simulink model "twa_parallel_pc104"  (R2016a)
settings: Solver=ode8  StartTime=0.0  StopTime=inf  FixedStep=dt  RelTol=1e-3
PreLoadFcn:
  | addpath('d:\Projects\TwistedWireActuator\TWA_parallel_control\init_func')
InitFcn:
  | init_main_twa
  | init_scopes
  | init_twa_homing
  | init_twa_wires
undefined symbols (not defined in the file or in its folder): b_in_w, dt, enc_res_vec, f_in_w, gear_rat_vec, Kd, Kd_mu, Ki, Ki_mu, Kp, Kp_mu, m_in_w, meas_flex_pos, N_velocity, p_in_m, pid_mode, qmacro_nom, res_rate_param, reset_integ, Signed, t_in_w, twa_gamma, twa_offset, use_twa, vel_filter_coeffs, velmex_pitch, wire_delta, wire_rad
libraries: xpcsensoraylib x7, slrtlib x6, simulink x4, dspswit3 x1
CloseFcn:
  | rtwprivate ssgencode ModelCloseRequest acrochordidae_v1
settings Model: Creator=Roger  LastModifiedBy=ahronoez
settings SolverCC: EnableConcurrentExecution=on
settings DataIOCC: SaveFormat=StructureWithTime  SignalLoggingSaveFormat=ModelDataLogs
settings OptimizationCC: BlockReduction=off  OptimizeBlockIOStorage=off  BufferReuse=off  GlobalBufferReuse=off  ExpressionFolding=off  ExpressionDepthLimit=2147483647  LocalBlockOutputs=off  InitFltsAndDblsToZero=on
settings DebuggingCC: UnderspecifiedInitializationDetection=Classic  MergeDetectMultiDrivingBlocksExec=none  SolverPrmCheckMsg=warning  FcnCallInpInsideContextMsg=UseLocalSettings  StateNameClashWarn=warning
settings HardwareCC: ProdBitPerPointer=32  ProdLargestAtomicFloat=None  ProdWordSize=32  ProdLongLongMode=on  ProdHWDeviceType=Generic->32-bit x86 compatible
settings ModelReferenceCC: PropagateSignalLabelsOutOfModel=off
settings SFSimCC: SimParseCustomCode=off
settings RTWCC: SystemTargetFile=slrt.tlc  TLCOptions=-aSLRTFTZOFF=1  TemplateMakefile=slrt_default_tmf  Description=Simulink Real-Time  GenerateReport=on  RTWCompilerOptimization=Custom  RTWCustomCompilerOptimizations=/arch-IA32
settings SimulinkRealTimeCC: xPCisDownloadable=off
settings ConfigComp: CovModelRefEnable=Off

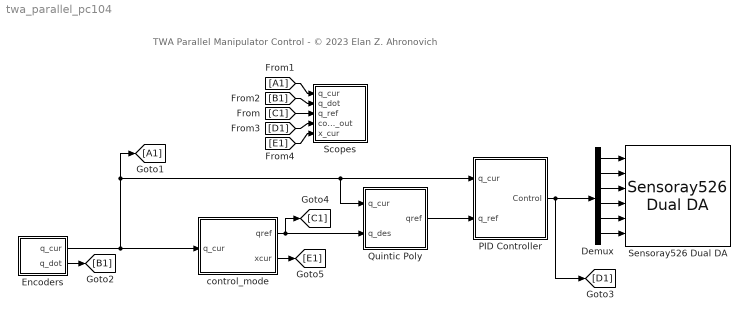
== system twa_parallel_pc104 ==
  note: TWA Parallel Manipulator Control - © 2023 Elan Z. Ahronovich
  Demux : Demux  Outputs=6
  Encoders : Subsystem
  PID Controller : Subsystem
  Quintic Poly : Subsystem
  Scopes : Subsystem
  "Sensoray526 Dual DA " : xpcsensoraylib/D//A/Sensoray526 Dual DA   channel1=[1 2 3 4]  reset1=[0]  initial1=[0]  channel2=[1 2]  reset2=[0]  initial2=[0]  sampletime=dt  baseaddress1=0x2c0  baseaddress2=0x340
  control_mode : Subsystem
  wires:
  PID Controller/1(Control) -> [D1], Demux/1
  Demux/1 -> "Sensoray526 Dual DA "/1
  Demux/2 -> "Sensoray526 Dual DA "/2
  Demux/3 -> "Sensoray526 Dual DA "/3
  Demux/4 -> "Sensoray526 Dual DA "/4
  Demux/5 -> "Sensoray526 Dual DA "/5
  Demux/6 -> "Sensoray526 Dual DA "/6
  Encoders/1(q_cur) -> PID Controller/1(q_cur), Quintic Poly/1(q_cur), [A1], control_mode/1(q_cur)
  Encoders/2(q_dot) -> [B1]
  Quintic Poly/1(qref) -> PID Controller/2(q_ref)
  [C1] -> Scopes/3(q_ref)
  [A1] -> Scopes/1(q_cur)
  [B1] -> Scopes/2(q_dot)
  [D1] -> Scopes/4(control_out)
  [E1] -> Scopes/5(x_cur)
  control_mode/1(qref) -> Quintic Poly/2(q_des), [C1]
  control_mode/2(xcur) -> [E1]

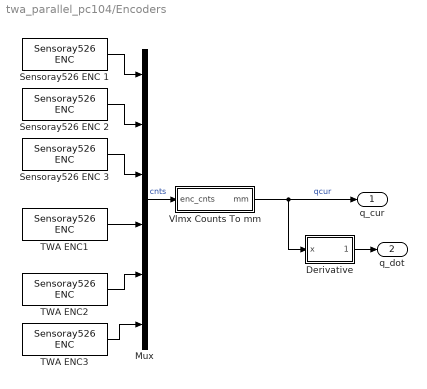
== system twa_parallel_pc104/Encoders ==
  Derivative : Subsystem
  Mux : Mux  Inputs=6
  Sensoray526 ENC 1 : xpcsensoraylib/Encoder/Sensoray526 ENC   channel=1  index=None  resetval=0  initval=0  range=Signed +-2^23  speed=4x  sampletime=dt  baseaddress=0x2c0
  Sensoray526 ENC 2 : xpcsensoraylib/Encoder/Sensoray526 ENC   channel=2  index=None  resetval=0  initval=0  range=Signed +-2^23  speed=4x  sampletime=dt  baseaddress=0x2c0
  Sensoray526 ENC 3 : xpcsensoraylib/Encoder/Sensoray526 ENC   channel=3  index=None  resetval=0  initval=0  range=Signed +-2^23  speed=4x  sampletime=dt  baseaddress=0x2c0
  TWA ENC1 : xpcsensoraylib/Encoder/Sensoray526 ENC   channel=4  index=None  resetval=0  initval=0  range=Signed +-2^23  speed=4x  sampletime=dt  baseaddress=0x2c0
  TWA ENC2 : xpcsensoraylib/Encoder/Sensoray526 ENC   channel=1  index=None  resetval=0  initval=0  range=Signed +-2^23  speed=4x  sampletime=dt  baseaddress=0x340
  TWA ENC3 : xpcsensoraylib/Encoder/Sensoray526 ENC   channel=2  index=None  resetval=0  initval=0  range=Signed +-2^23  speed=4x  sampletime=dt  baseaddress=0x340
  Vlmx Counts To mm : Subsystem
  q_cur : Outport
  q_dot : Outport  Port=2
  wires:
  Sensoray526 ENC 1/1 -> Mux/1
  Sensoray526 ENC 2/1 -> Mux/2
  Sensoray526 ENC 3/1 -> Mux/3
  Vlmx Counts To mm/1(mm) -> Derivative/1(x), q_cur/1  "qcur"
  Mux/1 -> Vlmx Counts To mm/1(enc_cnts)  "cnts"
  Derivative/1(x_dot) -> q_dot/1
  TWA ENC1/1 -> Mux/4
  TWA ENC2/1 -> Mux/5
  TWA ENC3/1 -> Mux/6

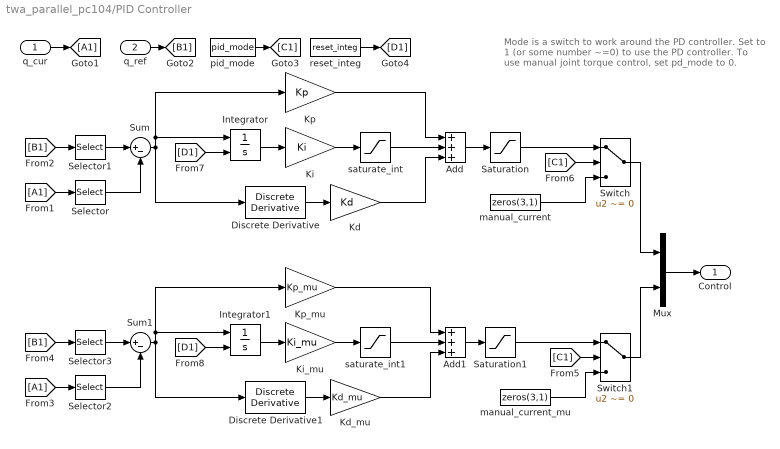
== system twa_parallel_pc104/PID Controller ==
  note: Mode is a switch to work around the PD controller.
      | Set to 1 (or some number ~=0) to use the PD
      | controller. To use manual joint torque control, set
      | pd_mode to 0.
  q_cur : Inport
  q_ref : Inport  Port=2
  Add : Sum  Inputs=+++
  Add1 : Sum  Inputs=+++
  Discrete Derivative : simulink/Discrete/Discrete Derivative  gainval=1.0  ICPrevScaledInput=0.0  InputProcessing=Inherited  OutMin=[]  OutMax=[]  OutDataType=fixdt(1, 16)  OutScaling=2^-10  DoSatur=off
  Discrete Derivative1 : simulink/Discrete/Discrete Derivative  gainval=1.0  ICPrevScaledInput=0.0  InputProcessing=Inherited  OutMin=[]  OutMax=[]  OutDataType=fixdt(1, 16)  OutScaling=2^-10  DoSatur=off
  Integrator : Integrator  ExternalReset=rising
  Integrator1 : Integrator  ExternalReset=rising
  Kd : Gain  Gain=Kd
  Kd_mu : Gain  Gain=Kd_mu
  Ki : Gain  Gain=Ki
  Ki_mu : Gain  Gain=Ki_mu
  Kp : Gain  Gain=Kp
  Kp_mu : Gain  Gain=Kp_mu
  Mux : Mux  Inputs=2
  Saturation : Saturate  UpperLimit=[10,10,10]  LowerLimit=-1*[10,10,10]  LinearizeAsGain=off
  Saturation1 : Saturate  UpperLimit=5*ones(3,1)  LowerLimit=-5*ones(3,1)  LinearizeAsGain=off
  Selector : Selector  InputPortWidth=6  IndexOptions=Index vector (dialog)  Indices=[1 2 3]  OutputSizes=1
  Selector1 : Selector  InputPortWidth=6  IndexOptions=Index vector (dialog)  Indices=[1 2 3]  OutputSizes=1
  Selector2 : Selector  InputPortWidth=6  IndexOptions=Index vector (dialog)  Indices=[4 5 6]  OutputSizes=1
  Selector3 : Selector  InputPortWidth=6  IndexOptions=Index vector (dialog)  Indices=[4 5 6]  OutputSizes=1
  Sum : Sum  Inputs=|+-
  Sum1 : Sum  Inputs=|+-
  Switch : Switch  Criteria=u2 ~= 0
  Switch1 : Switch  Criteria=u2 ~= 0
  manual_current : Constant  Value=zeros(3,1)  SampleTime=-1
  manual_current_mu : Constant  Value=zeros(3,1)  SampleTime=-1
  pid_mode : Constant  Value=pid_mode  SampleTime=-1
  reset_integ : Constant  Value=reset_integ  SampleTime=-1
  saturate_int : Saturate  UpperLimit=[5,5,5]  LowerLimit=-1*[5,5,5]  LinearizeAsGain=off
  saturate_int1 : Saturate  UpperLimit=2.5*ones(3,1)  LowerLimit=-2.5*ones(3,1)  LinearizeAsGain=off  SampleTime=dt
  Control : Outport
  wires:
  Kp/1 -> Add/1
  Kd/1 -> Add/3
  Add/1 -> Saturation/1
  Saturation/1 -> Switch/1
  manual_current/1 -> Switch/3
  Ki/1 -> saturate_int/1
  saturate_int/1 -> Add/2
  Discrete Derivative/1 -> Kd/1
  Integrator/1 -> Ki/1
  Sum/1 -> Kp/1, Integrator/1, Discrete Derivative/1
  Kp_mu/1 -> Add1/1
  Kd_mu/1 -> Add1/3
  Add1/1 -> Saturation1/1
  Saturation1/1 -> Switch1/1
  manual_current_mu/1 -> Switch1/3
  Ki_mu/1 -> saturate_int1/1
  saturate_int1/1 -> Add1/2
  Discrete Derivative1/1 -> Kd_mu/1
  Integrator1/1 -> Ki_mu/1
  Sum1/1 -> Kp_mu/1, Integrator1/1, Discrete Derivative1/1
  q_cur/1 -> [A1]
  q_ref/1 -> [B1]
  [A1] -> Selector/1
  [B1] -> Selector1/1
  [A1] -> Selector2/1
  [B1] -> Selector3/1
  pid_mode/1 -> [C1]
  [C1] -> Switch1/2
  [C1] -> Switch/2
  Mux/1 -> Control/1
  Switch/1 -> Mux/1
  Switch1/1 -> Mux/2
  Selector1/1 -> Sum/1
  Selector/1 -> Sum/2
  Selector3/1 -> Sum1/1
  Selector2/1 -> Sum1/2
  reset_integ/1 -> [D1]
  [D1] -> Integrator/2
  [D1] -> Integrator1/2

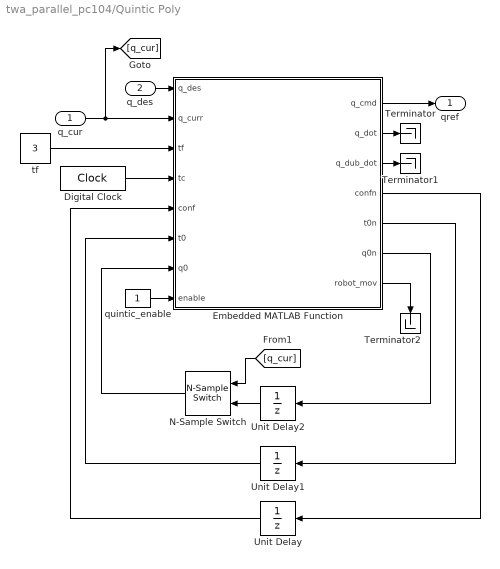
== system twa_parallel_pc104/Quintic Poly ==
  q_cur : Inport
  q_des : Inport  Port=2
  Digital Clock : DigitalClock  SampleTime=dt
  Embedded MATLAB Function : MATLAB Function  TreatAsAtomicUnit=on
  N-Sample Switch : dspswit3/N-Sample Switch  N=1  reset=off  TriggerType=Rising edge  Ts=dt
  Terminator : Terminator
  Terminator1 : Terminator
  Terminator2 : Terminator
  Unit Delay : UnitDelay  SampleTime=-1
  Unit Delay1 : UnitDelay  SampleTime=-1
  Unit Delay2 : UnitDelay  InitialCondition=zeros(6,1)  SampleTime=-1
  quintic_enable : Constant  SampleTime=-1
  tf : Constant  Value=3  SampleTime=-1
  qref : Outport
  wires:
  Embedded MATLAB Function/4(confn) -> Unit Delay/1
  Unit Delay/1 -> Embedded MATLAB Function/5(conf)
  Embedded MATLAB Function/5(t0n) -> Unit Delay1/1
  Embedded MATLAB Function/6(q0n) -> Unit Delay2/1
  Unit Delay1/1 -> Embedded MATLAB Function/6(t0)
  Digital Clock/1 -> Embedded MATLAB Function/4(tc)
  q_des/1 -> Embedded MATLAB Function/1(q_des)
  tf/1 -> Embedded MATLAB Function/3(tf)
  quintic_enable/1 -> Embedded MATLAB Function/8(enable)
  Embedded MATLAB Function/2(q_dot) -> Terminator/1
  Embedded MATLAB Function/3(q_dub_dot) -> Terminator1/1
  N-Sample Switch/1 -> Embedded MATLAB Function/7(q0)
  Unit Delay2/1 -> N-Sample Switch/2
  [q_cur] -> N-Sample Switch/1
  Embedded MATLAB Function/7(robot_mov) -> Terminator2/1
  Embedded MATLAB Function/1(q_cmd) -> qref/1
  q_cur/1 -> Embedded MATLAB Function/2(q_curr), [q_cur]

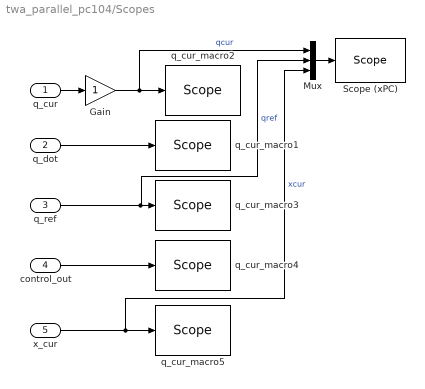
== system twa_parallel_pc104/Scopes ==
  q_cur : Inport
  q_dot : Inport  Port=2
  q_ref : Inport  Port=3
  control_out : Inport  Port=4
  x_cur : Inport  Port=5
  Gain : Gain
  Mux : Mux  Inputs=3
  "Scope (xPC) " : slrtlib/Displays and Logging/Scope   scopeno=6  scopetype=File  autostart=off  viewmode=Graphical redraw  formatstr='%15.6f'  grid=on  ylimits=[0,0]  nosamples=3  noprepostsamples=0  interleave=1  triggermode=FreeRun  triggersignal=1  trigsignalfromport=off  triggerlevel=0.0  triggerslope=Either  triggerscope=1  triggersample=0  filename=robot.dat  mode=Lazy  writesize=512  autorestart=on  dynamicfilemode=off  maxwritefilesize=512*1024^2
  q_cur_macro1 : slrtlib/Displays and Logging/Scope   scopeno=2  scopetype=Target  autostart=on  viewmode=Numerical  formatstr=qd_format  grid=on  ylimits=[0,0]  nosamples=25  noprepostsamples=0  interleave=1  triggermode=FreeRun  triggersignal=1  trigsignalfromport=off  triggerlevel=0.0  triggerslope=Either  triggerscope=1  triggersample=0  filename=data.dat  mode=Lazy  writesize=512  autorestart=off  dynamicfilemode=off  maxwritefilesize=512*1024^2
  q_cur_macro2 : slrtlib/Displays and Logging/Scope   scopeno=1  scopetype=Target  autostart=on  viewmode=Numerical  formatstr=q_format  grid=on  ylimits=[0,0]  nosamples=3  noprepostsamples=0  interleave=1  triggermode=FreeRun  triggersignal=1  trigsignalfromport=off  triggerlevel=0.0  triggerslope=Either  triggerscope=1  triggersample=0  filename=data.dat  mode=Lazy  writesize=512  autorestart=off  dynamicfilemode=off  maxwritefilesize=512*1024^2
  q_cur_macro3 : slrtlib/Displays and Logging/Scope   scopeno=3  scopetype=Target  autostart=on  viewmode=Numerical  formatstr=qdes_format  grid=on  ylimits=[0,0]  nosamples=25  noprepostsamples=0  interleave=1  triggermode=FreeRun  triggersignal=1  trigsignalfromport=off  triggerlevel=0.0  triggerslope=Either  triggerscope=1  triggersample=0  filename=data.dat  mode=Lazy  writesize=512  autorestart=off  dynamicfilemode=off  maxwritefilesize=512*1024^2
  q_cur_macro4 : slrtlib/Displays and Logging/Scope   scopeno=4  scopetype=Target  autostart=on  viewmode=Numerical  formatstr=qcmd_format  grid=on  ylimits=[0,0]  nosamples=25  noprepostsamples=0  interleave=1  triggermode=FreeRun  triggersignal=1  trigsignalfromport=off  triggerlevel=0.0  triggerslope=Either  triggerscope=1  triggersample=0  filename=data.dat  mode=Lazy  writesize=512  autorestart=off  dynamicfilemode=off  maxwritefilesize=512*1024^2
  q_cur_macro5 : slrtlib/Displays and Logging/Scope   scopeno=5  scopetype=Target  autostart=on  viewmode=Numerical  formatstr=xcur_format  grid=on  ylimits=[0,0]  nosamples=25  noprepostsamples=0  interleave=1  triggermode=FreeRun  triggersignal=1  trigsignalfromport=off  triggerlevel=0.0  triggerslope=Either  triggerscope=1  triggersample=0  filename=data.dat  mode=Lazy  writesize=512  autorestart=off  dynamicfilemode=off  maxwritefilesize=512*1024^2
  wires:
  q_ref/1 -> Mux/2, q_cur_macro3/1  "qref"
  control_out/1 -> q_cur_macro4/1
  x_cur/1 -> Mux/3, q_cur_macro5/1  "xcur"
  q_dot/1 -> q_cur_macro1/1
  q_cur/1 -> Gain/1
  Gain/1 -> Mux/1, q_cur_macro2/1  "qcur"
  Mux/1 -> "Scope (xPC) "/1

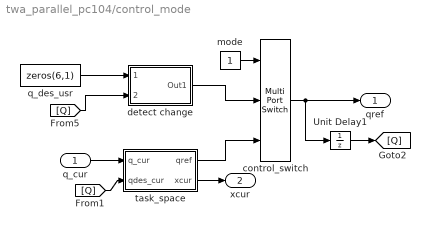
== system twa_parallel_pc104/control_mode ==
  q_cur : Inport
  Unit Delay1 : UnitDelay  InitialCondition=zeros(6,1)  SampleTime=-1
  control_switch : MultiPortSwitch  Inputs=2  DiagnosticForDefault=Warning
  detect change : Subsystem
  mode : Constant  SampleTime=-1
  q_des_usr : Constant  Value=zeros(6,1)  SampleTime=-1
  task_space : Subsystem
  qref : Outport
  xcur : Outport  Port=2
  wires:
  mode/1 -> control_switch/1
  control_switch/1 -> Unit Delay1/1, qref/1
  [Q] -> detect change/2(q_des_cur)
  detect change/1(Out1) -> control_switch/2
  q_des_usr/1 -> detect change/1(q_des_usr)
  q_cur/1 -> task_space/1(q_cur)
  task_space/2(xcur) -> xcur/1
  Unit Delay1/1 -> [Q]
  [Q] -> task_space/2(qdes_cur)
  task_space/1(qref) -> control_switch/3

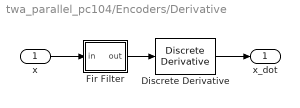
== system twa_parallel_pc104/Encoders/Derivative ==
  x : Inport
  Discrete Derivative : simulink/Discrete/Discrete Derivative  gainval=1.0  ICPrevScaledInput=0.0  InputProcessing=Inherited  OutMin=[]  OutMax=[]  OutDataType=fixdt(1, 16)  OutScaling=2^-10  DoSatur=off
  Fir Filter : Subsystem
  x_dot : Outport
  wires:
  Discrete Derivative/1 -> x_dot/1
  x/1 -> Fir Filter/1(in)
  Fir Filter/1(out) -> Discrete Derivative/1

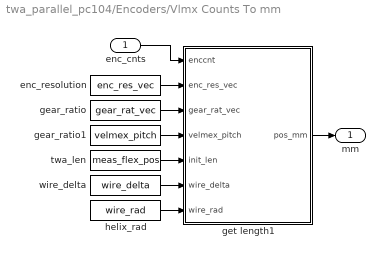
== system twa_parallel_pc104/Encoders/Vlmx Counts To mm ==
  enc_cnts : Inport
  enc_resolution : Constant  Value=enc_res_vec  SampleTime=-1
  gear_ratio : Constant  Value=gear_rat_vec  SampleTime=-1
  gear_ratio1 : Constant  Value=velmex_pitch  SampleTime=-1
  get length1 : MATLAB Function  TreatAsAtomicUnit=on
  helix_rad : Constant  Value=wire_rad  SampleTime=-1
  twa_len : Constant  Value=meas_flex_pos  SampleTime=-1
  wire_delta : Constant  Value=wire_delta  SampleTime=-1
  mm : Outport
  wires:
  helix_rad/1 -> get length1/7(wire_rad)
  wire_delta/1 -> get length1/6(wire_delta)
  twa_len/1 -> get length1/5(init_len)
  enc_resolution/1 -> get length1/2(enc_res_vec)
  gear_ratio/1 -> get length1/3(gear_rat_vec)
  enc_cnts/1 -> get length1/1(enccnt)
  get length1/1(pos_mm) -> mm/1
  gear_ratio1/1 -> get length1/4(velmex_pitch)

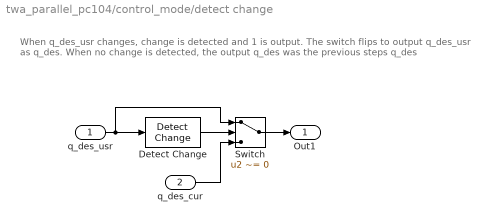
== system twa_parallel_pc104/control_mode/detect change ==
  note: When q_des_usr changes, change is detected and 1 is output.
      | The switch flips to output q_des_usr as q_des. When no change is detected, the output
      | q_des was the previous steps q_des
  q_des_usr : Inport
  q_des_cur : Inport  Port=2
  Detect Change : simulink/Logic and Bit Operations/Detect Change  vinit=zeros(6,1)  InputProcessing=Inherited  OutDataTypeStr=uint8
  Switch : Switch  Criteria=u2 ~= 0
  Out1 : Outport
  wires:
  Detect Change/1 -> Switch/2
  q_des_usr/1 -> Switch/1, Detect Change/1
  Switch/1 -> Out1/1
  q_des_cur/1 -> Switch/3

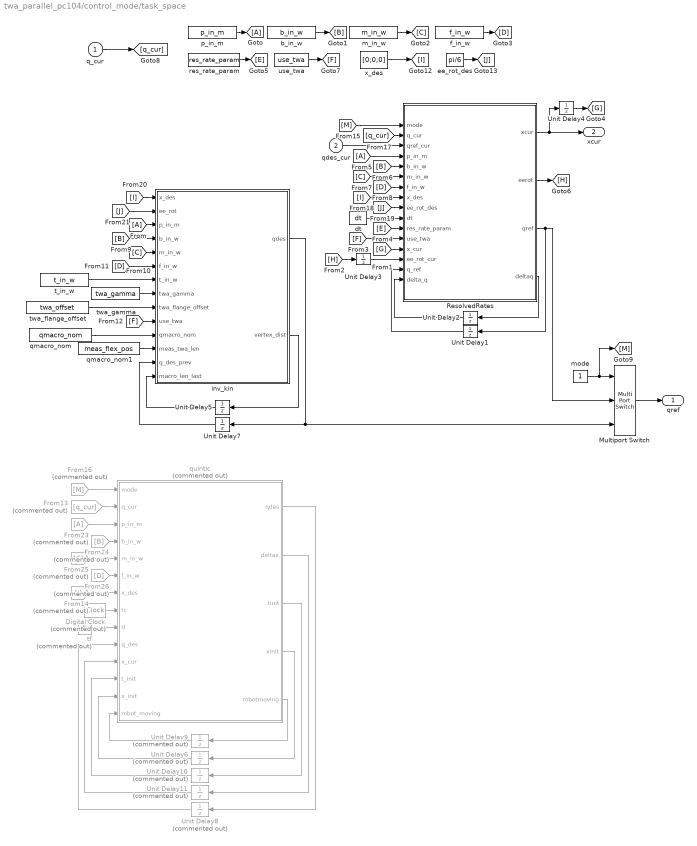
== system twa_parallel_pc104/control_mode/task_space ==
  q_cur : Inport
  qdes_cur : Inport  Port=2
  Digital Clock : DigitalClock  Commented=on  SampleTime=dt
  From13 : From  Commented=on  GotoTag=q_cur
  From14 : From  Commented=on  GotoTag=I
  From16 : From  Commented=on  GotoTag=M
  From23 : From  Commented=on
  From24 : From  Commented=on  GotoTag=B
  From25 : From  Commented=on  GotoTag=C
  From26 : From  Commented=on  GotoTag=D
  Multiport Switch : MultiPortSwitch  Inputs=2  DiagnosticForDefault=Warning
  ResolvedRates : MATLAB Function  TreatAsAtomicUnit=on
  Unit Delay1 : UnitDelay  InitialCondition=[0;0;0;0;0;0]  SampleTime=-1
  Unit Delay10 : UnitDelay  Commented=on  SampleTime=dt
  Unit Delay11 : UnitDelay  Commented=on  InitialCondition=[0;0;0]  SampleTime=dt
  Unit Delay2 : UnitDelay  InitialCondition=[0;0;0;0;0;0]  SampleTime=-1
  Unit Delay3 : UnitDelay  InitialCondition=pi/6  SampleTime=-1
  Unit Delay4 : UnitDelay  InitialCondition=[0;0;0]  SampleTime=-1
  Unit Delay5 : UnitDelay  InitialCondition=qmacro_nom  SampleTime=-1
  Unit Delay6 : UnitDelay  Commented=on  InitialCondition=[0;0;0]  SampleTime=dt
  Unit Delay7 : UnitDelay  InitialCondition=[0;0;0;0;0;0]  SampleTime=-1
  Unit Delay8 : UnitDelay  Commented=on  InitialCondition=zeros(6,1)  SampleTime=dt
  Unit Delay9 : UnitDelay  Commented=on  SampleTime=dt
  b_in_w : Constant  Value=b_in_w  SampleTime=-1
  dt : Constant  Value=dt  SampleTime=-1
  ee_rot_des : Constant  Value=pi/6  SampleTime=-1
  f_in_w : Constant  Value=f_in_w  SampleTime=-1
  inv_kin : MATLAB Function  TreatAsAtomicUnit=on
  m_in_w : Constant  Value=m_in_w  SampleTime=-1
  mode : Constant  SampleTime=-1
  p_in_m : Constant  Value=p_in_m  SampleTime=-1
  qmacro_nom : Constant  Value=qmacro_nom  SampleTime=-1
  qmacro_nom1 : Constant  Value=meas_flex_pos  SampleTime=-1
  quintic : MATLAB Function  Commented=on  TreatAsAtomicUnit=on
  res_rate_param : Constant  Value=res_rate_param  SampleTime=-1
  t_in_w : Constant  Value=t_in_w  SampleTime=-1
  tf : Constant  Commented=on  Value=5  SampleTime=dt
  twa_flange_offset : Constant  Value=twa_offset  SampleTime=-1
  twa_gamma : Constant  Value=twa_gamma  SampleTime=-1
  use_twa : Constant  Value=use_twa  SampleTime=-1
  x_des : Constant  Value=[0;0;0]  SampleTime=-1
  qref : Outport
  xcur : Outport  Port=2
  wires:
  p_in_m/1 -> [A]
  b_in_w/1 -> [B]
  m_in_w/1 -> [C]
  f_in_w/1 -> [D]
  dt/1 -> ResolvedRates/10(dt)
  qdes_cur/1 -> ResolvedRates/3(qref_cur)
  Unit Delay1/1 -> ResolvedRates/15(q_ref)
  ResolvedRates/3(qref) -> Unit Delay1/1, Multiport Switch/2
  [E] -> ResolvedRates/11(res_rate_param)
  res_rate_param/1 -> [E]
  ResolvedRates/2(eerot) -> [H]
  [H] -> Unit Delay3/1
  ResolvedRates/1(xcur) -> Unit Delay4/1, xcur/1
  [F] -> ResolvedRates/12(use_twa)
  use_twa/1 -> [F]
  ResolvedRates/4(deltaq) -> Unit Delay2/1
  Unit Delay2/1 -> ResolvedRates/16(delta_q)
  [A] -> inv_kin/3(p_in_m)
  [B] -> inv_kin/4(b_in_w)
  [C] -> inv_kin/5(m_in_w)
  [D] -> inv_kin/6(f_in_w)
  q_cur/1 -> [q_cur]
  [q_cur] -> ResolvedRates/2(q_cur)
  x_des/1 -> [I]
  ee_rot_des/1 -> [J]
  [I] -> ResolvedRates/8(x_des)
  [J] -> ResolvedRates/9(ee_rot_des)
  [I] -> inv_kin/1(x_des)
  [J] -> inv_kin/2(ee_rot)
  twa_gamma/1 -> inv_kin/8(twa_gamma)
  twa_flange_offset/1 -> inv_kin/9(twa_flange_offset)
  t_in_w/1 -> inv_kin/7(t_in_w)
  [F] -> inv_kin/10(use_twa)
  Multiport Switch/1 -> qref/1
  inv_kin/1(qdes) -> Multiport Switch/3, Unit Delay7/1
  Unit Delay7/1 -> inv_kin/13(q_des_prev)
  qmacro_nom/1 -> inv_kin/11(qmacro_nom)
  Unit Delay4/1 -> [G]
  Unit Delay3/1 -> ResolvedRates/14(ee_rot_cur)
  [G] -> ResolvedRates/13(x_cur)
  [A] -> ResolvedRates/4(p_in_m)
  [B] -> ResolvedRates/5(b_in_w)
  [C] -> ResolvedRates/6(m_in_w)
  [D] -> ResolvedRates/7(f_in_w)
  qmacro_nom1/1 -> inv_kin/12(meas_twa_len)
  inv_kin/2(vertex_dist) -> Unit Delay5/1
  Unit Delay5/1 -> inv_kin/14(macro_len_last)
  mode/1 -> [M], Multiport Switch/1
  [M] -> ResolvedRates/1(mode)
  From14/1 -> quintic/7(x_des)
  From23/1 -> quintic/3(p_in_m)
  From25/1 -> quintic/5(m_in_w)
  From24/1 -> quintic/4(b_in_w)
  From26/1 -> quintic/6(f_in_w)
  Digital Clock/1 -> quintic/8(tc)
  tf/1 -> quintic/9(tf)
  quintic/4(xinit) -> Unit Delay6/1
  quintic/5(robotmoving) -> Unit Delay9/1
  Unit Delay6/1 -> quintic/13(x_init)
  Unit Delay9/1 -> quintic/14(robot_moving)
  quintic/3(tinit) -> Unit Delay10/1
  Unit Delay10/1 -> quintic/12(t_init)
  quintic/2(deltax) -> Unit Delay11/1
  Unit Delay11/1 -> quintic/11(x_cur)
  quintic/1(qdes) -> Unit Delay8/1
  Unit Delay8/1 -> quintic/10(q_des)
  From13/1 -> quintic/2(q_cur)
  From16/1 -> quintic/1(mode)

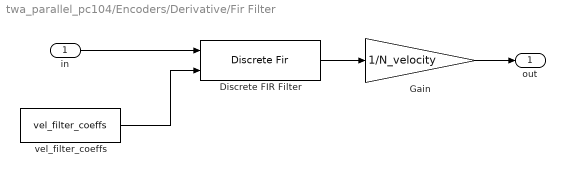
== system twa_parallel_pc104/Encoders/Derivative/Fir Filter ==
  in : Inport
  Discrete FIR Filter : DiscreteFir  CoefSource=Input port  AccumDataTypeStr=Inherit: Same as product output
      settings: InputPortMap=u0,u1
  Gain : Gain  Gain=1/N_velocity
  vel_filter_coeffs : Constant  Value=vel_filter_coeffs  SampleTime=-1
  out : Outport
  wires:
  Discrete FIR Filter/1 -> Gain/1
  vel_filter_coeffs/1 -> Discrete FIR Filter/2
  Gain/1 -> out/1
  in/1 -> Discrete FIR Filter/1

== matlab function twa_parallel_pc104/control_mode/task_space/ResolvedRates ==
  data: xcur output; eerot output; mode input; q_cur input; qref_cur input; p_in_m input; b_in_w input; m_in_w input; f_in_w input; qref output; x_des input; ee_rot_des input; dt input; res_rate_param input; use_twa input; x_cur input; ee_rot_cur input; q_ref input; delta_q input; deltaq output
% using resolved rates with redundacny resolution to solve robot position
% elan ahronovich 08/2024

function [xcur,eerot,qref,deltaq] = redResRate(mode,q_cur,qref_cur,...
    p_in_m,b_in_w,m_in_w,f_in_w,x_des,ee_rot_des,...
    dt,res_rate_param,use_twa,x_cur,ee_rot_cur,q_ref,delta_q)

% initialize
qref = qref_cur;
eerot = ee_rot_cur;
deltaq = delta_q;

% if using inv kin to control robot position its a safe assumption from the
% perspective of resolved rates that the current position of the ee is the 
% requested desired position. This helps keep the resolved rates updated
% with the current robot position without relying on the resolved rates to 
% solve for it which will accumulate error over some time
if mode == 2
    xcur = x_des;
else
    xcur = x_cur;
end

% axis for jacobian definitions
z0 = [0 0 1]';

% rotation matrix
r_cur = [cos(ee_rot_cur) -sin(ee_rot_cur) 0;sin(ee_rot_cur) cos(ee_rot_cur) 0;0 0 1];

% moving platform vertex locations
p_in_w = x_cur*ones(1,3) + r_cur*p_in_m;

%% instantaneous direct kinematics jacobian
% vector from base vertex to moving platform vertex
n1hat = (p_in_w(:,1)-b_in_w(:,1))./norm(b_in_w(:,1) - p_in_w(:,1));
n2hat = (p_in_w(:,2)-b_in_w(:,2))./norm(b_in_w(:,2) - p_in_w(:,2));
n3hat = (p_in_w(:,3)-b_in_w(:,3))./norm(b_in_w(:,3) - p_in_w(:,3));

a13 = z0'*(cross(r_cur*p_in_m(:,1),n1hat));
a23 = z0'*(cross(r_cur*p_in_m(:,2),n2hat));
a33 = z0'*(cross(r_cur*p_in_m(:,3),n3hat));

idk_jac = [n1hat(1,1) n1hat(2,1) a13; ...
    n2hat(1,1) n2hat(2,1) a23; ...
    n3hat(1,1) n3hat(2,1) a33];

%% instantaneous inverse kinematics jacobian
% micro actuator (TWA) lengths
q1_mu = norm(b_in_w(:,1) - m_in_w(:,1));
q2_mu = norm(b_in_w(:,2) - m_in_w(:,2));
q3_mu = norm(b_in_w(:,3) - m_in_w(:,3));

% vector from base vertex to twa motor attachment point
l1_hat = (m_in_w(:,1) - b_in_w(:,1)) ./ norm(m_in_w(:,1) - b_in_w(:,1));
l2_hat = (m_in_w(:,2) - b_in_w(:,2)) ./ norm(m_in_w(:,2) - b_in_w(:,2));
l3_hat = (m_in_w(:,3) - b_in_w(:,3)) ./ norm(m_in_w(:,3) - b_in_w(:,3));

% distance from micro actuator attachmnet point (m_i) to flexure rotation
%center (f_i)
a1 = norm(m_in_w(:,1) - f_in_w(:,1));
a2 = norm(m_in_w(:,2) - f_in_w(:,2));
a3 = norm(m_in_w(:,3) - f_in_w(:,3));

% distance from flexure rotation center (f_i) to base vertex
c1 = norm(b_in_w(:,1)-f_in_w(:,1));
c2 = norm(b_in_w(:,2)-f_in_w(:,2));
c3 = norm(b_in_w(:,3)-f_in_w(:,3));

% term to paramterize angle between a_i and qimu, delta
h1 = (c1^2 - a1^2 - q1_mu^2)/(-2*a1*q1_mu);
h2 = (c2^2 - a2^2 - q2_mu^2)/(-2*a2*q2_mu);
h3 = (c3^2 - a3^2 - q3_mu^2)/(-2*a3*q3_mu);

% time derivatives
h1dot = (4*a1*q1_mu^2 + (c1^2 - a1^2 - q1_mu^2)*2*a1) / (4*a1^2*q1_mu^2);
h2dot = (4*a2*q2_mu^2 + (c2^2 - a2^2 - q2_mu^2)*2*a2) / (4*a2^2*q2_mu^2);
h3dot = (4*a3*q3_mu^2 + (c3^2 - a3^2 - q3_mu^2)*2*a3) / (4*a3^2*q3_mu^2);

e1 = n1hat' * l1_hat + q1_mu*h1dot/sqrt(1-h1^2) * n1hat' * cross(z0,l1_hat);
e2 = n2hat' * l2_hat + q2_mu*h2dot/sqrt(1-h2^2) * n2hat' * cross(z0,l2_hat);
e3 = n3hat' * l3_hat + q3_mu*h3dot/sqrt(1-h3^2) * n3hat' * cross(z0,l3_hat);

% micro motion instantaneous inverse kinematics jacobian
b_mu = [e1 0 0;...
    0 e2 0;...
    0 0 e3];

% macro motion instantaneous inverse kinematics jacobian
b_m = eye(3);

% combined macro-micro motion IIK jacobian
iik_jac = [b_m,b_mu];

% positional error
p_del = norm(x_des - x_cur);

% positional error direction vector
if p_del ~= 0
    p_ep_hat = (x_des-x_cur)/p_del;
else
    p_ep_hat = zeros(3,1);
end

%*
% This can probably be replaced with scalar angular difference that will
% always bout about me = [0 0 1]'
%*

% desired orientation angle rotation matrix and error roation matrix
r_des = [cos(ee_rot_des) -sin(ee_rot_des) 0;sin(ee_rot_des) cos(ee_rot_des) 0;0 0 1];
r_cur = [cos(ee_rot_cur) -sin(ee_rot_cur) 0;sin(ee_rot_cur) cos(ee_rot_cur) 0;0 0 1];
r_del = r_des * r_cur';

% orientational error angle and axis
theta_e = acos((trace(r_del)-1)/2);

% orientational error axis
if theta_e ~= 0
    me = (1/(2*sin(theta_e)))*[r_del(3,2)-r_del(2,3);...
        r_del(1,3)-r_del(3,1);...
        r_del(2,1)-r_del(1,2)];
else
    me = z0;
end

% error thresholds
p_eps = res_rate_param(1,1);
w_eps = res_rate_param(2,1);
p_eps_mu = res_rate_param(1,2);
w_eps_mu = res_rate_param(2,2);

% linear velocity
vmax = res_rate_param(3,1);
vmin = res_rate_param(4,1);
vmax_mu = res_rate_param(3,2);
vmin_mu = res_rate_param(4,2);

% rotational velocity
wmax = res_rate_param(5,1);
wmin = res_rate_param(6,1);
wmax_mu = res_rate_param(5,2);
wmin_mu = res_rate_param(6,2);

% convergence radius multiplier
p_lambda = res_rate_param(7,1);
w_lambda = res_rate_param(8,1);
p_lambda_mu = res_rate_param(7,2);
w_lambda_mu = res_rate_param(8,2);

if mode == 1
    if theta_e > w_eps || p_del > p_eps
        % linear velocity multiplier
        if p_del ~=0
            if p_del/p_eps <= p_lambda
                vdot = vmin + (((vmax-vmin)*(p_del-p_eps))/(p_eps*(p_lambda-1)));
            else
                vdot = vmax;
            end
        else
            vdot = 0;
        end
        
        % angular velocity multiplier
        if theta_e ~= 0
            if theta_e/w_eps <= w_lambda && theta_e ~= 0
                wdot = wmin + (((wmax-wmin)*(theta_e-w_eps))/(w_eps*(w_lambda-1)));
            else
                wdot = wmax;
            end
        else
            wdot = 0;
        end
        
        % xdot_des components
        v = vdot * p_ep_hat;
        w = wdot * me;
        
        % jacobian weight matrix for macro actuator preference
        w_mat = diag([ones(1,3),1e10*ones(1,3)]);
        
        % construct jacobian
        full_jac = (w_mat\iik_jac') / (iik_jac/w_mat*iik_jac') * idk_jac;
        
        % qdot des using inverse kinematics with redundancy
        qdot = full_jac * [v(1:2);w(3)];
        
        % new desired q values
        deltaq = qdot * dt;

        qref = q_ref + deltaq;
        
        % integrate current position
        xcur = x_cur + v * dt;
        eerot = ee_rot_cur + w(3) * dt;
        % now that the macro motion has converged we can use micro actuators
    elseif theta_e > w_eps_mu || p_del > p_eps_mu
        if use_twa
            %         qdes = qdes_cur;
            %         xcur = x_cur;
            %         eerot = ee_rot_cur;
            % same as macro, only iterate twa length if they have arrived at
            % last desired location
            % linear velocity multiplier
            if p_del ~=0
                if p_del/p_eps_mu <= p_lambda_mu
                    vdot = vmin_mu + (((vmax_mu-vmin_mu)*...
                        (p_del-p_eps_mu))/(p_eps_mu*(p_lambda_mu-1)));
                else
                    vdot = vmax_mu;
                end
            else
                vdot = 0;
            end
            
            % angular velocity multiplier
            if theta_e ~= 0
                if theta_e/w_eps_mu <= w_lambda_mu && theta_e ~= 0
                    wdot = wmin_mu + (((wmax_mu - wmin_mu)*...
                        (theta_e - w_eps_mu))/(w_eps_mu*(w_lambda_mu-1)));
                else
                    wdot = wmax_mu;
                end
            else
                wdot = 0;
            end
            
            % xdot_des components
            v = vdot * p_ep_hat;
            w = wdot * me;
            
            % jacobian weight matrix for micro actuator preference
            w_mat = diag([1e10*ones(1,3),ones(1,3)]);
            
            % construct jacobian
            full_jac = (w_mat\iik_jac') / (iik_jac/w_mat*iik_jac') * idk_jac;
            
            % qdot des using inverse kinematics with redundancy
            qdot = full_jac * [v(1:2,1);w(3,1)];
            
            % new desired q values
            deltaq = qdot * dt;
            qref = q_ref + deltaq;
            
            % integrate current position
            xcur = x_cur + (dt*v);
            eerot = ee_rot_cur + w(3) * dt;
        end
    end
end

end

== matlab function twa_parallel_pc104/control_mode/task_space/quintic ==
  data: qdes output; mode input; q_cur input; p_in_m input; b_in_w input; m_in_w input; f_in_w input; x_des input; tc input; tf input; q_des input; x_cur input; t_init input; x_init input; deltax output; tinit output; xinit output; robot_moving input; robotmoving output
% using resolved rates with redundacny resolution to solve robot position
% elan ahronovich 08/2024

function [qdes,deltax,tinit,xinit,robotmoving] = quintic(mode,q_cur,...
    p_in_m,b_in_w,m_in_w,f_in_w,x_des,...
    tc,tf,q_des,x_cur,t_init,x_init,robot_moving)

% initialize
qdes = q_des;
deltax = x_cur;
tinit = t_init;
xinit = x_init;
robotmoving = robot_moving;

if mode == 3; do_quintic = 1; else do_quintic =0; end

% axis for jacobian definitions
z0 = [0 0 1]';

% rotation matrix
ee_rot_cur = pi/6;
r_cur = [cos(ee_rot_cur) -sin(ee_rot_cur) 0;sin(ee_rot_cur) cos(ee_rot_cur) 0;0 0 1];

% moving platform vertex locations
p_in_w = x_cur*ones(1,3) + r_cur*p_in_m;

%% instantaneous direct kinematics jacobian
% vector from base vertex to moving platform vertex
n1hat = (p_in_w(:,1)-b_in_w(:,1))./norm(b_in_w(:,1) - p_in_w(:,1));
n2hat = (p_in_w(:,2)-b_in_w(:,2))./norm(b_in_w(:,2) - p_in_w(:,2));
n3hat = (p_in_w(:,3)-b_in_w(:,3))./norm(b_in_w(:,3) - p_in_w(:,3));

a13 = z0'*(cross(r_cur*p_in_m(:,1),n1hat));
a23 = z0'*(cross(r_cur*p_in_m(:,2),n2hat));
a33 = z0'*(cross(r_cur*p_in_m(:,3),n3hat));

idk_jac = [n1hat(1,1) n1hat(2,1) a13; ...
    n2hat(1,1) n2hat(2,1) a23; ...
    n3hat(1,1) n3hat(2,1) a33];

%% instantaneous inverse kinematics jacobian
% micro actuator (TWA) lengths
q1_mu = norm(b_in_w(:,1) - m_in_w(:,1));
q2_mu = norm(b_in_w(:,2) - m_in_w(:,2));
q3_mu = norm(b_in_w(:,3) - m_in_w(:,3));

% vector from base vertex to twa motor attachment point
l1_hat = (m_in_w(:,1) - b_in_w(:,1)) ./ norm(m_in_w(:,1) - b_in_w(:,1));
l2_hat = (m_in_w(:,2) - b_in_w(:,2)) ./ norm(m_in_w(:,2) - b_in_w(:,2));
l3_hat = (m_in_w(:,3) - b_in_w(:,3)) ./ norm(m_in_w(:,3) - b_in_w(:,3));

% distance from micro actuator attachmnet point (m_i) to flexure rotation
%center (f_i)
a1 = norm(m_in_w(:,1) - f_in_w(:,1));
a2 = norm(m_in_w(:,2) - f_in_w(:,2));
a3 = norm(m_in_w(:,3) - f_in_w(:,3));

% distance from flexure rotation center (f_i) to base vertex
c1 = norm(b_in_w(:,1)-f_in_w(:,1));
c2 = norm(b_in_w(:,2)-f_in_w(:,2));
c3 = norm(b_in_w(:,3)-f_in_w(:,3));

% term to paramterize angle between a_i and qimu, delta
h1 = (c1^2 - a1^2 - q1_mu^2)/(-2*a1*q1_mu);
h2 = (c2^2 - a2^2 - q2_mu^2)/(-2*a2*q2_mu);
h3 = (c3^2 - a3^2 - q3_mu^2)/(-2*a3*q3_mu);

% time derivatives
h1dot = (4*a1*q1_mu^2 + (c1^2 - a1^2 - q1_mu^2)*2*a1) / (4*a1^2*q1_mu^2);
h2dot = (4*a2*q2_mu^2 + (c2^2 - a2^2 - q2_mu^2)*2*a2) / (4*a2^2*q2_mu^2);
h3dot = (4*a3*q3_mu^2 + (c3^2 - a3^2 - q3_mu^2)*2*a3) / (4*a3^2*q3_mu^2);

e1 = n1hat' * l1_hat + q1_mu*h1dot/sqrt(1-h1^2) * n1hat' * cross(z0,l1_hat);
e2 = n2hat' * l2_hat + q2_mu*h2dot/sqrt(1-h2^2) * n2hat' * cross(z0,l2_hat);
e3 = n3hat' * l3_hat + q3_mu*h3dot/sqrt(1-h3^2) * n3hat' * cross(z0,l3_hat);

% micro motion instantaneous inverse kinematics jacobian
b_mu = [e1 0 0;...
    0 e2 0;...
    0 0 e3];

% macro motion instantaneous inverse kinematics jacobian
b_m = eye(3);

% combined macro-micro motion IIK jacobian
iik_jac = [b_m,b_mu];

% positional error
p_del = x_des - x_init;
w_del = norm(x_des(3,1) - x_init(3,1));

%
if do_quintic && norm(p_del) > 0
    if robot_moving
        t = tc - t_init;
        if t < tf
            eta = t/tf;
            a3 = 10*eta^3;
            a4 = -15*eta^4;
            a5 = 6*eta^5;
            
            % apply quintic polynomial on task space
            deltax = x_init + p_del*(a3+a4+a5);
            
            % redundancy weight matrix favoring velmex up to 50 microns
            % from destination
            if norm(p_del) > 0.050
                w_mat = diag([ones(1,3),1e10*ones(1,3)]);
               macro_motion = 1;
            else
                w_mat = diag([ones(1,3),1e10*ones(1,3)]);
                macro_motion = 0;
            end
            
            % construct jacobian
            full_jac = (w_mat\iik_jac') / (iik_jac/w_mat*iik_jac') * idk_jac;
            
            % deltaq ~ J * deltax
            deltaq = full_jac * deltax;
            
            % new desired q values
            if macro_motion
                % new desired q values
                qdes(1:3,1) = deltaq(1:3,1);
                qdes(4:6,1) = q_cur(4:6,1);
            else
                qdes(4:6,1) = deltaq(4:6,1);
                qdes(1:3,1) = q_cur(1:3,1);
            end
        else
            robotmoving = 0;
        end
    else
        qdes = q_cur;
        tinit = tc;
        xinit = x_cur;
        robotmoving = 1;
    end
end

end

== matlab function twa_parallel_pc104/Encoders/Vlmx Counts To mm/get length1 ==
  data: enccnt input; enc_res_vec input; gear_rat_vec input; velmex_pitch input; init_len input; wire_delta input; wire_rad input; pos_mm output
% this function converts encoder counts to mm
% elan ahronovich 09/2024

function pos_mm  = fcn(enccnt,enc_res_vec,gear_rat_vec,velmex_pitch,init_len,wire_delta,wire_rad)
% velmex slides
pos_mm1 = enccnt(1,1)*(1/enc_res_vec(1,1))*(1/gear_rat_vec(1,1))*velmex_pitch;
pos_mm2 = enccnt(2,1)*(1/enc_res_vec(2,1))*(1/gear_rat_vec(2,1))*velmex_pitch;
pos_mm3 = enccnt(3,1)*(1/enc_res_vec(3,1))*(1/gear_rat_vec(3,1))*velmex_pitch;

% twisted wire actuators
% convert counts to radians
theta_mu1 = enccnt(4,1)*(1/enc_res_vec(4,1))*(1/gear_rat_vec(4,1))*2*pi; %[radians]
theta_mu2 = enccnt(5,1)*(1/enc_res_vec(5,1))*(1/gear_rat_vec(5,1))*2*pi; %[radians]
theta_mu3 = enccnt(6,1)*(1/enc_res_vec(6,1))*(1/gear_rat_vec(6,1))*2*pi; %[radians]

% estimate length of helix. model cannot handle when motors return to zero
% for some reason, the motors will run off. force a constant solution for
% the length in this case
if theta_mu1 == 0
    twa_len1 = 0;
else
    twa_len1 = init_len(1,1)-sqrt(init_len(1,1)^2*(1+wire_delta(1,1))^2 - (theta_mu1^2*wire_rad(1,1)^2));
end

if theta_mu2 == 0
    twa_len2 = 0;
else
    twa_len2 = init_len(2,1)-sqrt(init_len(2,1)^2*(1+wire_delta(2,1))^2 - (theta_mu2^2*wire_rad(2,1)^2));
end

if theta_mu3 == 0
    twa_len3 = 0;
else
    twa_len3 = init_len(3,1)-sqrt(init_len(3,1)^2*(1+wire_delta(3,1))^2 - (theta_mu3^2*wire_rad(3,1)^2));
end

pos_mm = [pos_mm1;pos_mm2;pos_mm3;twa_len1;twa_len2;twa_len3];
end

== matlab function twa_parallel_pc104/control_mode/task_space/inv_kin ==
  data: qdes output; vertex_dist output; x_des input; ee_rot input; p_in_m input; b_in_w input; m_in_w input; f_in_w input; t_in_w input; twa_gamma input; twa_flange_offset input; use_twa input; qmacro_nom input; meas_twa_len input; q_des_prev input; macro_len_last input
% This function solves for the vertex positions of the base and moving
% platform for a given desired end effector position.
% elan ahronovich 07/2024

function [qdes,vertex_dist] = fcn(x_des,ee_rot,p_in_m,b_in_w,m_in_w,f_in_w,...
                                  t_in_w,twa_gamma,twa_flange_offset,use_twa,...
                                  qmacro_nom,meas_twa_len,q_des_prev,macro_len_last)

qdes = q_des_prev;
% des_micro_len = micro_len;

vertex_dist = macro_len_last;

% rotation matrix of moving frame about z-xis
rot_m2w = [cos(ee_rot) -sin(ee_rot) 0; sin(ee_rot) cos(ee_rot) 0; 0 0 1];

p_in_w = x_des*ones(1,3) + rot_m2w*p_in_m;

%%%%%%%%%%%%%%%%%%%%%%%%%%%%%%%%
%        Macro Actuator        %
%%%%%%%%%%%%%%%%%%%%%%%%%%%%%%%%

if ~use_twa
    vertex_dist = p_in_w - b_in_w;
    qdes(1,1) = norm(vertex_dist(:,1)) - norm(qmacro_nom(:,1));
    qdes(2,1) = norm(vertex_dist(:,2)) - norm(qmacro_nom(:,2));
    qdes(3,1) = norm(vertex_dist(:,3)) - norm(qmacro_nom(:,3));
end

%%%%%%%%%%%%%%%%%%%%%%%%%%%%%%%%
%       Micro Actuator         %
%%%%%%%%%%%%%%%%%%%%%%%%%%%%%%%%

if use_twa 
    % initial flexure bend
    beta_cmd = 0;
    
    % loop through each vertex
    for i = 1:3
        post_flex_angle = zeros(1,2);
        beta = zeros(1,2);
        
        % vector from flexure center to moving platform vertex
        rho_vec = p_in_w(:,i) - f_in_w(:,i);
        
        % distance between flexure and moving platform verteces
        rho = norm(rho_vec);
        
        % vector from flexure center to base vertex pre flexure rotation
        eta_vec = b_in_w(:,i) - f_in_w(:,i);
        
        % flexure angle at the start (e.g. 5 deg preload) in world frame
        pre_flex_angle = atan2(eta_vec(2,1),eta_vec(1,1));
        
        % magnitude of flexure swing-arm radius from flexure to base vertex
        eta = norm(eta_vec);
        
        % angle from world horizontal to the vector from the flexure
        % center to the platform vertex
        flexure_frame_rot_angle = atan2(rho_vec(2,1),rho_vec(1,1));
        
        % rotation matrix from flexure frame to world
        n = [0;0;1] ./ norm([0;0;1]);
        rot_f_2_w = expm(flexure_frame_rot_angle*[0 -n(3) n(2);n(3) 0 -n(1);n(2) n(1) 0]);
        
        % condition for acos solvability
        check = (norm(vertex_dist(:,i))^2-rho^2-eta^2)/(-2*rho*eta);
%         check = (des_macro_len(i,1)^2-rho^2-eta^2)/(-2*rho*eta);
        
        if check >= -1 && check <= 1
            % calculate angle between mf and fb vectors, lambda, with
            % law of cosines
            lambda = acos(check);
            
            % calculate flexed base vertex position for both elbow up
            % and down configurations in the flexure frame
            b_prime_in_f_dwn = eta*[cos(-lambda);sin(-lambda);0];
            b_prime_in_f_up = eta*[cos(lambda);sin(lambda);0];
            
            % vector from flexure center point to new base vertex location
            % rotated to world frame
            eta_prime_vec_dwn = rot_f_2_w*b_prime_in_f_dwn;
            eta_prime_vec_up = rot_f_2_w*b_prime_in_f_up;
            
            post_flex_angle(1,1) = atan2(eta_prime_vec_dwn(2,1),eta_prime_vec_dwn(1,1));
            post_flex_angle(1,2) = atan2(eta_prime_vec_up(2,1),eta_prime_vec_up(1,1));
            
            % determine if flex angle is within mechanical range
            for j = 1:2
                if pre_flex_angle < 0 && post_flex_angle(1,j) < 0
                    beta(1,j) = (-1*pre_flex_angle)-(-1*post_flex_angle(1,j));
                else
                    beta(1,j) = pre_flex_angle - post_flex_angle(1,j);
                end
                
                if beta(1,j) >= -4*pi/180 && beta(1,j) <= 4*pi/180
                    beta_cmd = beta(1,j);
                end
            end
        end
        
        % initial angle prior to flexure bend
        a = norm(f_in_w(:,i) - m_in_w(:,i));
        b = norm(f_in_w(:,i) - b_in_w(:,i));
        c = norm(m_in_w(:,i) - b_in_w(:,i));
        %c = init_twa_len(i,1);
        
        alpha =  acos((c^2 - a^2 - b^2)/(-2*a*b));
        delta = alpha - beta_cmd;
        
        % distance between base vertex and twa motor position after flex
        c_prime = sqrt(a^2 + b^2 - 2*a*b*cos(delta));
        
        % distance between flexure center of rotation and twa attachment
        d = norm(f_in_w(:,1) - t_in_w(:,1));        
        
        % required twa length to facilitate flexure bend
        des_micro_len = sqrt(a^2 + d^2 - 2*a*d*cos(delta - twa_gamma))...
                                - twa_flange_offset;
                            
        qdes(3+i,1) = meas_twa_len(i,1) - des_micro_len;
    end
end

== matlab function twa_parallel_pc104/Quintic Poly/Embedded MATLAB Function ==
  data: q_cmd output; q_des input; q_curr input; tf input; tc input; q_dot output; q_dub_dot output; conf input; confn output; t0 input; t0n output; q0n output; q0 input; enable input; robot_mov output
function [q_cmd,q_dot,q_dub_dot,confn,t0n,q0n,robot_mov] = fifth_order_p(q_des,q_curr,tf,tc,conf,t0,q0,enable)
% number of actuators
n = size(q_des,1);

robot_mov = 0;
eta = q_des - q0;

if enable
    if (eta)'*(eta) > 0
        % conf = 0 means that the 5th order poly
        % is not configured for the desired trajectory.
        % Therefore, the block is initialized.
        if conf == 0               
            q0n = q0;               
            t0n = tc;               
            confn = 1;
            q_cmd = q0;
            q_dot = zeros(n,1);
            q_dub_dot = zeros(n,1);
        else
            q0n = q0;
            t0n = t0;
            confn = conf;
            
            % 5th order polynomial
            a0 = q0;
            a4 = -15*(eta);
            a3 = -2/3 * a4;
            a5 = -2/5 * a4;
            t = tc-t0;
            tau = t/tf;
            
            if t < tf
                robot_mov = 1;
                q_cmd = a0 + a3 * tau^3 + a4 * tau^4 + a5 * tau^5;
                q_dot = 3*a3*t^2/tf^3 + 4*a4*t^3/tf^4 + 5*a5*t^4/tf^5;
                q_dub_dot = 6*a3*t/tf^3 + 12*a4*t^2/tf^4 + 20*a5*t^3/tf^5;
            else
                q_cmd = q_des;
                q_dot = zeros(n,1);
                q_dub_dot = zeros(n,1);
                q0n = q_des;
            end
        end
    else
        q_cmd = q_des;
        q_dot = zeros(n,1);
        q_dub_dot = zeros(n,1);
        confn = 0;
        q0n = q0;
        t0n = t0;
    end
else
    % Configuration space is not used (pdot = 0).
    q_cmd = q_des;
    q_dot = zeros(n,1);
    q_dub_dot = zeros(n,1);       % However we do want to record the current
    confn = 0;                  % position in order to be ready as soon
    t0n = tc;                   % as the enable becomes 1.
    q0n = q_curr;
end
%------------------------------------------------------------------------
